simulink model "Activity_3_Sim"  (R2022a)
settings: Solver=VariableStepAuto  StartTime=0.0  StopTime=10.0  RelTol=1e-3
values from neighbouring files (symbols this model uses):
  Sine_Amplitude_i = 1    [Run_Sim_Activity_3.m]
  Sine_Freq_i = 100    [Run_Sim_Activity_3.m]
settings Model: Creator=chadw  LastModifiedBy=chadw

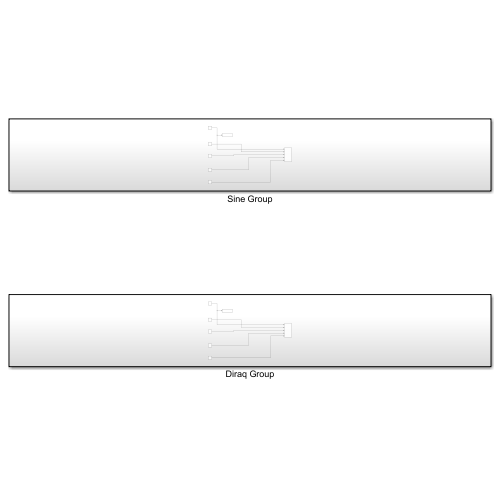
[thumbnail: Simulink's stored preview of the top-level diagram]
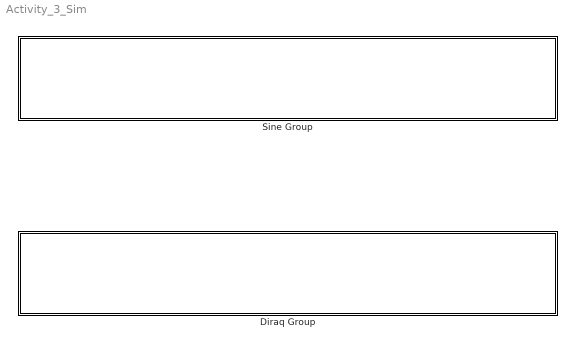
== system Activity_3_Sim ==
  Diraq Group : Subsystem
  Sine Group : Subsystem

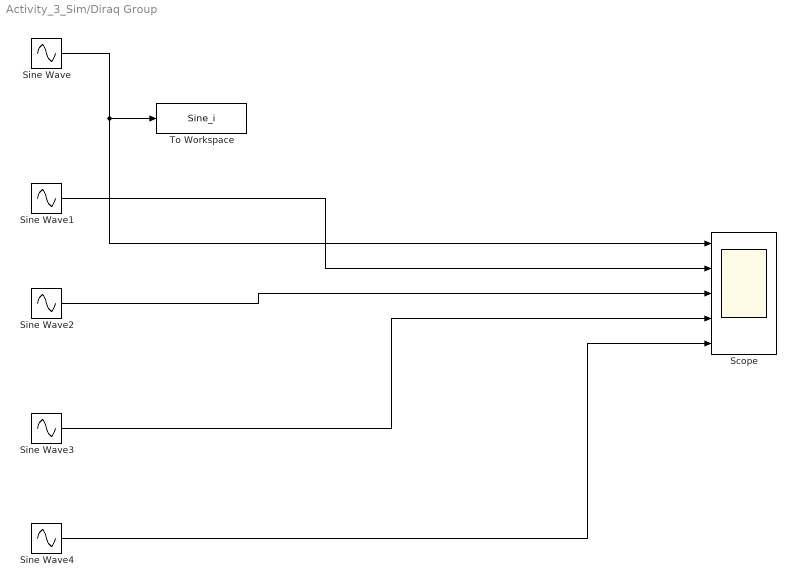
== system Activity_3_Sim/Diraq Group ==
  Scope : Scope  NumInputPorts=5
  Sine Wave : Sin  Amplitude=Sine_Amplitude_i  Frequency=Sine_Freq_i  SampleTime=0
  Sine Wave{1..4} (4 alike) : Sin  SampleTime=0
  To Workspace : ToWorkspace  VariableName=Sine_i  SampleTime=-1
  wires:
  Sine Wave3/1 -> Scope/4
  Sine Wave1/1 -> Scope/2
  Sine Wave2/1 -> Scope/3
  Sine Wave4/1 -> Scope/5
  Sine Wave/1 -> Scope/1, To Workspace/1

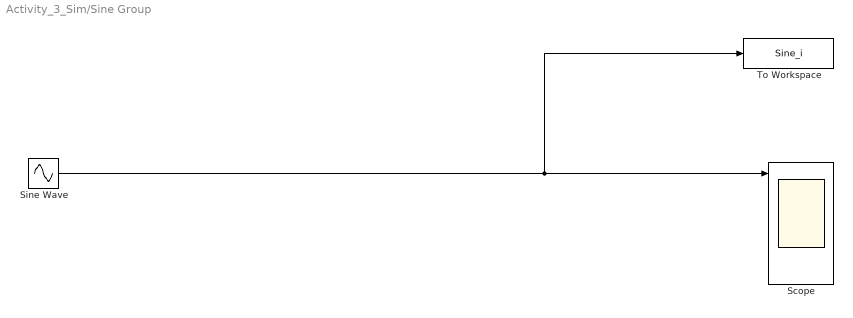
== system Activity_3_Sim/Sine Group ==
  Scope : Scope  NumInputPorts=5
  Sine Wave : Sin  Amplitude=Sine_Amplitude_i  Frequency=Sine_Freq_i  SampleTime=0
  To Workspace : ToWorkspace  VariableName=Sine_i  SampleTime=-1
  wires:
  Sine Wave/1 -> To Workspace/1, Scope/1
